simulink model "model3"  (R2021b)
settings: Solver=VariableStepAuto  StartTime=0.0  StopTime=100.0  RelTol=1e-3
settings Model: Creator=Clement_Wu  LastModifiedBy=Clement_Wu

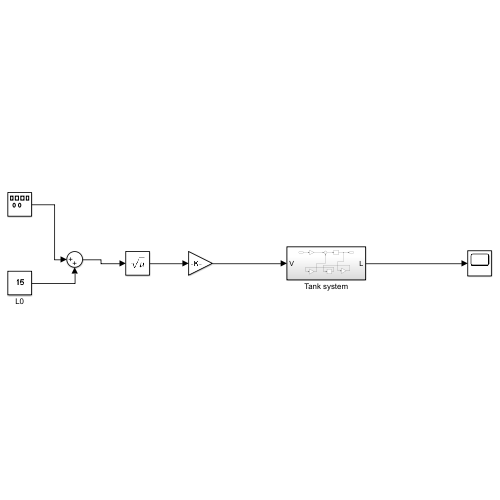
[thumbnail: Simulink's stored preview of the top-level diagram]
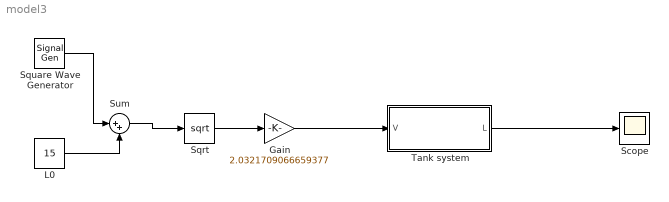
== system model3 ==
  Gain : Gain  Gain=2.0321709066659377
  L0 : Constant  Value=15
  Scope : Scope
  Sqrt : Sqrt  SaturateOnIntegerOverflow=on
  Square Wave Generator : SignalGenerator  WaveForm=square  Units=rad/sec
  Sum : Sum  Inputs=|++
  Tank system : Subsystem
  wires:
  Tank system/1(L) -> Scope/1
  Gain/1 -> Tank system/1(V)
  Sqrt/1 -> Gain/1
  Square Wave Generator/1 -> Sum/1
  L0/1 -> Sum/2
  Sum/1 -> Sqrt/1

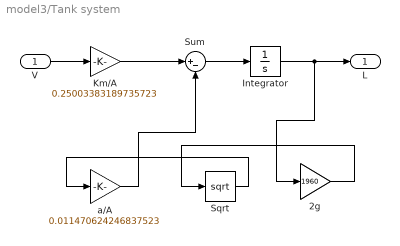
== system model3/Tank system ==
  V : Inport
  2g : Gain  Gain=1960
  Integrator : Integrator
  Km/A : Gain  Gain=0.25003383189735723
  Sqrt : Sqrt  SaturateOnIntegerOverflow=on
  Sum : Sum  Inputs=|+-
  a/A : Gain  Gain=0.011470624246837523
  L : Outport
  wires:
  Integrator/1 -> 2g/1, L/1
  2g/1 -> Sqrt/1
  Sqrt/1 -> a/A/1
  V/1 -> Km/A/1
  Km/A/1 -> Sum/1
  a/A/1 -> Sum/2
  Sum/1 -> Integrator/1
